simulink library "lib_fuel_converter"  (Simulink 4.00)
undefined symbols (not defined in the file): acc_mech_eff, acc_mech_pwr, acc_mech_trq, air_cp, amb_tmp, cyc_mph, ex_gas_cp, fc_acc_mass, fc_base_mass, fc_c2i_th_cond, fc_c_init_tmp, fc_cl2h_eff, fc_CO2_to_FUELgps, fc_cold, fc_cold_tmp, fc_cp, fc_ct_trq, fc_emisv, fc_ext_sarea, fc_fuel_den, fc_fuel_lhv, fc_h2x_th_cond, fc_h_air_flow, fc_h_cp, fc_h_init_tmp, fc_hood_emisv, fc_hood_sarea, fc_i2x_th_cond, fc_i_init_tmp, fc_inertia, fc_map_spd, fc_map_trq, fc_max_trq, fc_nn_model_name, fc_pwr_scale, fc_spd_scale, fc_trq_scale, fc_tstat, fc_x_init_tmp, fd_ratio, gb_num_init, gb_ratio, pow, vc_idle_spd, vc_key_on, veh_glider_mass, veh_mass, wh_radius
libraries: lib_fuel_converter x6, lib_etc x4
(part 3 of 4)

== system lib_fuel_converter/fuel converter  <fc> for series/spinning up or spinning down/effect of inertia (Nm) ==
  note: if initial speed is >0 and it is the
      | first time step ignore inertial loads
      | tm:2/6/01
  req'd spd (rad/s) : Inport  Port=1  LatchInput=off
  prev spd : Inport  Port=2  LatchInput=off
  Clock : Clock
      settings: DisplayTime=off  Decimation=10
  Constant : Constant  Value=fc_inertia
  Constant1 : Constant  Value=cyc_mph(1,2)
  Logical Operator : Logic  Operator=NAND  Inputs=2
  Logical Operator1 : Logic  Operator=NOT  Inputs=2
  Memory : Memory  X0=-0.1  InheritSampleTime=off
      settings: RTWStateStorageClass=Auto
  Memory1 : Memory  X0=0  InheritSampleTime=off
      settings: RTWStateStorageClass=Auto
  Product1 : Product  Inputs=**/*  Multiplication=Element-wise(.*)  SaturateOnIntegerOverflow=on
  Sum : Sum  Inputs=+-  SaturateOnIntegerOverflow=on
  Sum1 : Sum  Inputs=+-  SaturateOnIntegerOverflow=on
  (Nm) : Outport  Port=1  InitialOutput=0
  wires:
  Logical Operator1/1 -> Logical Operator/2
  Memory1/1 -> Logical Operator1/1
  Constant1/1 -> Logical Operator/1
  Logical Operator/1 -> Product1/4
  Sum/1 -> Product1/2
  Sum1/1 -> Product1/3
  req'd spd (rad/s)/1 -> Sum/1
  prev spd/1 -> Sum/2
  Product1/1 -> (Nm)/1
  Memory/1 -> Sum1/2
  Clock/1 -> Memory1/1, Memory/1, Sum1/1
  Constant/1 -> Product1/1

== system lib_fuel_converter/fuel converter  <fc> for series/spinning up or spinning down/just started spin-down/spin-up ==
  state : Inport  Port=1  LatchInput=off
  Logical Operator : Logic  Operator=AND  Inputs=2
  Logical Operator1 : Logic  Operator=NOT  Inputs=1
  Memory1 : Memory  X0=(cyc_mph(1,2)==0)  InheritSampleTime=off
      settings: RTWStateStorageClass=Auto
  trigger : Outport  Port=1  InitialOutput=0
  wires:
  Memory1/1 -> Logical Operator1/1
  Logical Operator1/1 -> Logical Operator/2
  Logical Operator/1 -> trigger/1
  state/1 -> Logical Operator/1, Memory1/1

== system lib_fuel_converter/fuel converter  <fc> for series/spinning up or spinning down/no-lag Reset Integrator ==
  in_1 : Inport  Port=1  LatchInput=off
  in_2 : Inport  Port=2  LatchInput=off
  in_3 : Inport  Port=3  LatchInput=off
  Constant : Constant  Value=0
  Memory : Memory  Orientation=left  X0=initval  InheritSampleTime=off
      settings: RTWStateStorageClass=Auto
  Product : Product  Inputs=2  Multiplication=Element-wise(.*)  SaturateOnIntegerOverflow=on
  Sum : Sum  Inputs=++  SaturateOnIntegerOverflow=on
  Switch : Switch  Threshold=eps
  dt : Subsystem  Orientation=down
      settings: RTWFcnNameOpts=Auto  RTWFileNameOpts=Auto
  in_2==0 : RelationalOperator  Operator===
  out_1 : Outport  Port=1  InitialOutput=0
  wires:
  in_3/1 -> Switch/3
  in_2/1 -> in_2==0/1
  in_1/1 -> Product/2
  dt/1(out_1) -> Product/1
  Product/1 -> Sum/2
  Memory/1 -> Sum/1
  Sum/1 -> Switch/1
  Switch/1 -> out_1/1, Memory/1
  in_2==0/1 -> Switch/2
  Constant/1 -> in_2==0/2

== system lib_fuel_converter/fuel converter  <fc> prius/providing trq (+ive or -ive)/accessories (Nm) ==
  w_APU : Inport  Port=1  LatchInput=off
  (Nm) : Product  Inputs=*/  Multiplication=Element-wise(.*)  SaturateOnIntegerOverflow=on
  (W) : Product  Inputs=*/  Multiplication=Element-wise(.*)  SaturateOnIntegerOverflow=on
  Constant : Constant  Value=acc_mech_pwr
  Constant1 : Constant  Value=acc_mech_eff
  Constant2 : Constant  Orientation=down  Value=acc_mech_trq
  Constant3 : Constant  Orientation=left  Value=0
  Saturation : Saturate  UpperLimit=inf  LowerLimit=vc_idle_spd+eps  LinearizeAsGain=on
  Sum : Sum  Inputs=++  SaturateOnIntegerOverflow=on
  Switch : Switch  Threshold=eps
  key_on : Subsystem  Orientation=left  mask(Repeating table){@1=vc_key_on(:,1), @2=vc_key_on(:,2)}
      mask prompts: @1 "Time values:"; @2 "Output values:"
      mask help:
      | Repeating table.
      | Enter values of time and output for first cycle.
      mask init:
      | period = max(@1); t = @1; y = @2;
      settings: RTWFcnNameOpts=Auto  RTWFileNameOpts=Auto
      mask Help: Repeats cycle given in table. Time values should be monotonically increasing.
  T_acc : Outport  Port=1  InitialOutput=0
  wires:
  Saturation/1 -> (Nm)/2
  Switch/1 -> T_acc/1
  Constant3/1 -> Switch/3
  key_on/1(out_1) -> Switch/2
  Sum/1 -> Switch/1
  Constant2/1 -> Sum/1
  (Nm)/1 -> Sum/2
  (W)/1 -> (Nm)/1
  w_APU/1 -> Saturation/1
  Constant1/1 -> (W)/2
  Constant/1 -> (W)/1

== system lib_fuel_converter/fuel converter  <fc> prius/providing trq (+ive or -ive)/effect of inertia (Nm) ==
  req'd spd (rad/s) : Inport  Port=1  LatchInput=off
  prev spd : Inport  Port=2  LatchInput=off
  Clock : Clock
      settings: DisplayTime=off  Decimation=10
  Constant : Constant  Value=fc_inertia
  Memory : Memory  X0=-0.1  InheritSampleTime=off
      settings: RTWStateStorageClass=Auto
  Product1 : Product  Inputs=**/  Multiplication=Element-wise(.*)  SaturateOnIntegerOverflow=on
  Sum : Sum  Inputs=+-  SaturateOnIntegerOverflow=on
  Sum1 : Sum  Inputs=+-  SaturateOnIntegerOverflow=on
  (Nm) : Outport  Port=1  InitialOutput=0
  wires:
  Sum/1 -> Product1/2
  Sum1/1 -> Product1/3
  req'd spd (rad/s)/1 -> Sum/1
  prev spd/1 -> Sum/2
  Product1/1 -> (Nm)/1
  Memory/1 -> Sum1/2
  Clock/1 -> Memory/1, Sum1/1
  Constant/1 -> Product1/1

== system lib_fuel_converter/fuel converter  <fc> prius/providing trq (+ive or -ive)/enforce engine limits ==
  req'd engine trq (Nm) : Inport  Port=1  LatchInput=off
  req'd engine spd (rad/s) : Inport  Port=2  LatchInput=off
  Block NOTES : Subsystem
      settings: RTWFcnNameOpts=Auto  RTWFileNameOpts=Auto
      mask Display: disp('Block\nNOTES')
  MinMax : MinMax  Function=min  Inputs=2
  MinMax1 : MinMax  Function=max  Inputs=2
  Relational Operator : RelationalOperator  Operator=~=
  Saturation : Saturate  UpperLimit=max(fc_map_spd)*fc_spd_scale  LowerLimit=0  LinearizeAsGain=on
  T_closed throttle : Subsystem
      settings: RTWFcnNameOpts=Auto  RTWFileNameOpts=Auto
  T_max : Subsystem
      settings: RTWFcnNameOpts=Auto  RTWFileNameOpts=Auto
  clutch disengaged1 : RelationalOperator  Operator=~=
  limited engine brake trq (Nm) : Outport  Port=1
  limited engine spd (rad/s) : Outport  Port=2
  tag scope: fc_spd_limited=global, fc_trq_limited=global
  wires:
  T_closed throttle/1(T_closed throttle) -> MinMax1/2
  Relational Operator/1 -> [fc_spd_limited]
  MinMax/1 -> MinMax1/1
  T_max/1(T_max) -> MinMax/2
  clutch disengaged1/1 -> [fc_trq_limited]
  MinMax1/1 -> limited engine brake trq (Nm)/1, clutch disengaged1/2
  req'd engine trq (Nm)/1 -> MinMax/1, clutch disengaged1/1
  Saturation/1 -> T_closed throttle/1(w_APU), T_max/1(w_APU), limited engine spd (rad/s)/1, Relational Operator/2
  req'd engine spd (rad/s)/1 -> Saturation/1, Relational Operator/1

== system lib_fuel_converter/configurable subsystems/fuel use and EO emis/HOT engine maps /Block NOTES ==
  note: This block determines the fully hot fuel use, engine-out emissions output rates, exhaust gas mass flow rate,
      | and engine-out exhaust gas temperature as a function of engine output torque and speed.
      | The engine maps (except for exhaust gas temperature) can be scaled using variables fc_spd_scale and
      |  fc_trq_scale; it is recommended that scaling values outside the range of 0.85 to 1.15 be used CAREFULLY.

== system lib_fuel_converter/configurable subsystems/fuel use and EO emis/HOT engine maps /CO (g/s) ==
  x0 : Inport  Port=1  LatchInput=off
  y0 : Inport  Port=2  LatchInput=off
  Mux : Mux  Inputs=2
      settings: DisplayOption=none
  S-function : S-Function  FunctionName=sftable2  Parameters=xindex, yindex, table  PortCounts=[]  SFunctionModules=''
  table out : Outport  Port=1  InitialOutput=0
  wires:
  y0/1 -> Mux/2
  S-function/1 -> table out/1
  x0/1 -> Mux/1
  Mux/1 -> S-function/1

== system lib_fuel_converter/configurable subsystems/fuel use and EO emis/HOT engine maps /HC (g/s) ==
  x0 : Inport  Port=1  LatchInput=off
  y0 : Inport  Port=2  LatchInput=off
  Mux : Mux  Inputs=2
      settings: DisplayOption=none
  S-function : S-Function  FunctionName=sftable2  Parameters=xindex, yindex, table  PortCounts=[]  SFunctionModules=''
  table out : Outport  Port=1  InitialOutput=0
  wires:
  y0/1 -> Mux/2
  S-function/1 -> table out/1
  x0/1 -> Mux/1
  Mux/1 -> S-function/1

== system lib_fuel_converter/configurable subsystems/fuel use and EO emis/HOT engine maps /MF,ex (g/s) ==
  x0 : Inport  Port=1  LatchInput=off
  y0 : Inport  Port=2  LatchInput=off
  Mux : Mux  Inputs=2
      settings: DisplayOption=none
  S-function : S-Function  FunctionName=sftable2  Parameters=xindex, yindex, table  PortCounts=[]  SFunctionModules=''
  table out : Outport  Port=1  InitialOutput=0
  wires:
  y0/1 -> Mux/2
  S-function/1 -> table out/1
  x0/1 -> Mux/1
  Mux/1 -> S-function/1

== system lib_fuel_converter/configurable subsystems/fuel use and EO emis/HOT engine maps /NOx (g/s) ==
  x0 : Inport  Port=1  LatchInput=off
  y0 : Inport  Port=2  LatchInput=off
  Mux : Mux  Inputs=2
      settings: DisplayOption=none
  S-function : S-Function  FunctionName=sftable2  Parameters=xindex, yindex, table  PortCounts=[]  SFunctionModules=''
  table out : Outport  Port=1  InitialOutput=0
  wires:
  y0/1 -> Mux/2
  S-function/1 -> table out/1
  x0/1 -> Mux/1
  Mux/1 -> S-function/1

== system lib_fuel_converter/configurable subsystems/fuel use and EO emis/HOT engine maps /O2 (g/s) ==
  x0 : Inport  Port=1  LatchInput=off
  y0 : Inport  Port=2  LatchInput=off
  Mux : Mux  Inputs=2
      settings: DisplayOption=none
  S-function : S-Function  FunctionName=sftable2  Parameters=xindex, yindex, table  PortCounts=[]  SFunctionModules=''
  table out : Outport  Port=1  InitialOutput=0
  wires:
  Mux/1 -> S-function/1
  x0/1 -> Mux/1
  S-function/1 -> table out/1
  y0/1 -> Mux/2

== system lib_fuel_converter/configurable subsystems/fuel use and EO emis/HOT engine maps /PM (g/s) ==
  x0 : Inport  Port=1  LatchInput=off
  y0 : Inport  Port=2  LatchInput=off
  Mux : Mux  Inputs=2
      settings: DisplayOption=none
  S-function : S-Function  FunctionName=sftable2  Parameters=xindex, yindex, table  PortCounts=[]  SFunctionModules=''
  table out : Outport  Port=1  InitialOutput=0
  wires:
  y0/1 -> Mux/2
  S-function/1 -> table out/1
  x0/1 -> Mux/1
  Mux/1 -> S-function/1

== system lib_fuel_converter/configurable subsystems/fuel use and EO emis/HOT engine maps /Tex,eo (C) ==
  x0 : Inport  Port=1  LatchInput=off
  y0 : Inport  Port=2  LatchInput=off
  Mux : Mux  Inputs=2
      settings: DisplayOption=none
  S-function : S-Function  FunctionName=sftable2  Parameters=xindex, yindex, table  PortCounts=[]  SFunctionModules=''
  table out : Outport  Port=1  InitialOutput=0
  wires:
  y0/1 -> Mux/2
  S-function/1 -> table out/1
  x0/1 -> Mux/1
  Mux/1 -> S-function/1

== system lib_fuel_converter/configurable subsystems/fuel use and EO emis/HOT engine maps /fuel (g/s) ==
  x0 : Inport  Port=1  LatchInput=off
  y0 : Inport  Port=2  LatchInput=off
  Mux : Mux  Inputs=2
      settings: DisplayOption=none
  S-function : S-Function  FunctionName=sftable2  Parameters=xindex, yindex, table  PortCounts=[]  SFunctionModules=''
  table out : Outport  Port=1  InitialOutput=0
  wires:
  y0/1 -> Mux/2
  S-function/1 -> table out/1
  x0/1 -> Mux/1
  Mux/1 -> S-function/1

== system lib_fuel_converter/configurable subsystems/fuel use and EO emis/fc temp/Block NOTES ==
  note: This block models the thermal behavior internal combustion engine (ICE).
      | Emphasis is on the coolant since this temperature is used to correct engine
      | fuel use.

== system lib_fuel_converter/configurable subsystems/fuel use and EO emis/fc temp/fc coolant ==
  Tcl : Inport  Port=1  LatchInput=off
  "Qfc_i " : Inport  Port=2  LatchInput=off
  Enable : EnablePort  StatesWhenEnabling=reset
  Constant : Constant  Value=fc_tstat
  Product1 : Product  Inputs=2  Multiplication=Element-wise(.*)  SaturateOnIntegerOverflow=on
  Qhtr : Fcn  Expr=fc_cl2h_eff*fc_h_air_flow*air_cp*(u - amb_tmp)
  Qi : Sum  Inputs=-+  SaturateOnIntegerOverflow=on
  Relational Operator : RelationalOperator  Operator=<=
  Qfc_rad : Outport  Port=1  OutputWhenDisabled=reset  InitialOutput=0
  Qfc_htr : Outport  Port=2  OutputWhenDisabled=reset  InitialOutput=0
  wires:
  Qi/1 -> Product1/2
  Qhtr/1 -> Qfc_htr/1, Qi/1
  "Qfc_i "/1 -> Qi/2
  Product1/1 -> Qfc_rad/1
  Constant/1 -> Relational Operator/1
  Relational Operator/1 -> Product1/1
  Tcl/1 -> Relational Operator/2, Qhtr/1

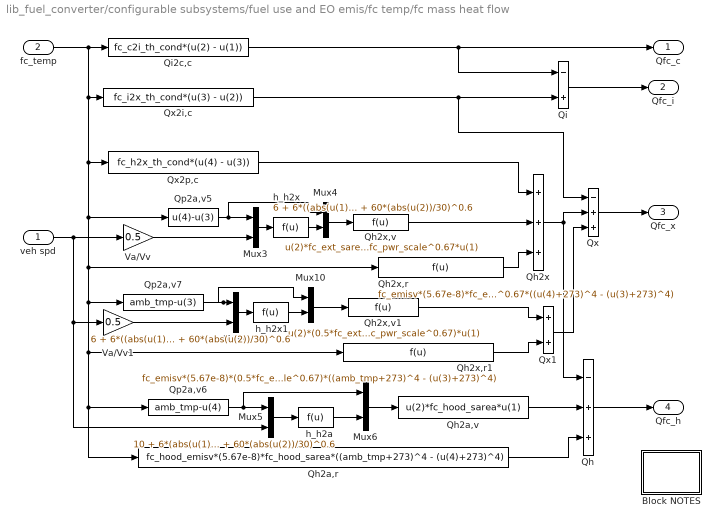
== system lib_fuel_converter/configurable subsystems/fuel use and EO emis/fc temp/fc mass heat flow ==
  veh spd : Inport  Port=1  LatchInput=off
  fc_temp : Inport  Port=2  LatchInput=off
  Block NOTES : Subsystem
      settings: RTWFcnNameOpts=Auto  RTWFileNameOpts=Auto
      mask Display: disp('Block\nNOTES')
  Mux{3..6,9..10} (6 alike) : Mux  Inputs=2
      settings: DisplayOption=none
  Qh : Sum  Inputs=-++  SaturateOnIntegerOverflow=on
  Qh2a,r : Fcn  Expr=fc_hood_emisv*(5.67e-8)*fc_hood_sarea*((amb_tmp+273)^4 - (u(4)+273)^4)
  Qh2a,v : Fcn  Expr=u(2)*fc_hood_sarea*u(1)
  Qh2x : Sum  Inputs=+++  SaturateOnIntegerOverflow=on
  Qh2x,r : Fcn  Expr=fc_emisv*(5.67e-8)*fc_ext_sarea*fc_pwr_scale^0.67*((u(4)+273)^4 - (u(3)+273)^4)
  Qh2x,r1 : Fcn  Expr=fc_emisv*(5.67e-8)*(0.5*fc_ext_sarea*fc_pwr_scale^0.67)*((amb_tmp+273)^4 - (u(3)+273)^4)
  Qh2x,v : Fcn  Expr=u(2)*fc_ext_sarea*fc_pwr_scale^0.67*u(1)
  Qh2x,v1 : Fcn  Expr=u(2)*(0.5*fc_ext_sarea*fc_pwr_scale^0.67)*u(1)
  Qi : Sum  Inputs=-+  SaturateOnIntegerOverflow=on
  Qi2c,c : Fcn  Expr=fc_c2i_th_cond*(u(2) - u(1))
  Qp2a,v5 : Fcn  Expr=u(4)-u(3)
  Qp2a,v6 : Fcn  Expr=amb_tmp-u(4)
  Qp2a,v7 : Fcn  Expr=amb_tmp-u(3)
  Qx : Sum  Inputs=-++  SaturateOnIntegerOverflow=on
  Qx1 : Sum  Inputs=++  SaturateOnIntegerOverflow=on
  Qx2i,c : Fcn  Expr=fc_i2x_th_cond*(u(3) - u(2))
  Qx2p,c : Fcn  Expr=fc_h2x_th_cond*(u(4) - u(3))
  Va/Vv : Gain  Gain=0.5  Multiplication=Element-wise(K.*u)  SaturateOnIntegerOverflow=on
  Va/Vv1 : Gain  Gain=0.5  Multiplication=Element-wise(K.*u)  SaturateOnIntegerOverflow=on
  h_h2a : Fcn  Expr=10 + 6*(abs(u(1))/1000)^0.3 + 60*(abs(u(2))/30)^0.6
  h_h2x : Fcn  Expr=6 + 6*((abs(u(1))/1000))^0.3 + 60*(abs(u(2))/30)^0.6
  h_h2x1 : Fcn  Expr=6 + 6*((abs(u(1))/1000))^0.3 + 60*(abs(u(2))/30)^0.6
  Qfc_c : Outport  Port=1
  Qfc_i : Outport  Port=2
  Qfc_x : Outport  Port=3
  Qfc_h : Outport  Port=4
  wires:
  Qh2x,r/1 -> Qh2x/3
  Qh2a,v/1 -> Qh/2
  Qh2a,r/1 -> Qh/3
  Qh2x,v1/1 -> Qx1/1
  Qh2x,r1/1 -> Qx1/2
  Qx2p,c/1 -> Qh2x/1
  Qh2x,v/1 -> Qh2x/2
  Qx1/1 -> Qx/3
  h_h2a/1 -> Mux6/2
  Qp2a,v6/1 -> Mux6/1, Mux5/1
  Mux5/1 -> h_h2a/1
  Mux6/1 -> Qh2a,v/1
  Qh/1 -> Qfc_h/1
  Qh2x/1 -> Qh/1, Qx/2
  Qx/1 -> Qfc_x/1
  Qi/1 -> Qfc_i/1
  Qx2i,c/1 -> Qx/1, Qi/2
  fc_temp/1 -> Qi2c,c/1, Qx2i,c/1, Qp2a,v5/1, Qh2x,r1/1, Qh2a,r/1, Qp2a,v6/1, Qp2a,v7/1, Qh2x,r/1, Qx2p,c/1
  Qi2c,c/1 -> Qi/1, Qfc_c/1
  Va/Vv/1 -> Mux3/2
  veh spd/1 -> Va/Vv1/1, Mux5/2, Va/Vv/1
  h_h2x/1 -> Mux4/2
  Qp2a,v5/1 -> Mux4/1, Mux3/1
  Mux3/1 -> h_h2x/1
  Mux4/1 -> Qh2x,v/1
  Va/Vv1/1 -> Mux9/2
  h_h2x1/1 -> Mux10/2
  Qp2a,v7/1 -> Mux10/1, Mux9/1
  Mux9/1 -> h_h2x1/1
  Mux10/1 -> Qh2x,v1/1

== system lib_fuel_converter/configurable subsystems/fuel use and EO emis/fc temp/old fc coolant  temp. (C) ==
  fc on? : Inport  Port=1  LatchInput=off
  veh spd : Inport  Port=2  LatchInput=off
  Block NOTES : Subsystem
      settings: RTWFcnNameOpts=Auto  RTWFileNameOpts=Auto
      mask Display: disp('Block\nNOTES')
  Mux : Mux  Inputs=4
      settings: DisplayOption=none
  TEC : Integrator  ExternalReset=none  InitialConditionSource=internal  InitialCondition=fc_i_init_tmp  LimitOutput=off  UpperSaturationLimit=inf  LowerSaturationLimit=-inf  ShowSaturationPort=off  ShowStatePort=off  AbsoluteTolerance=auto
  compute engine dT/dt : Fcn  Expr=1.1*u[1]*(-u[2]/218)*(95-u[4])+(1-u[1])*u[3]*(u[4]-amb_tmp)
  gamma (takes v as input) : Fcn  Expr=(-8.22e-5*u+8.09e-6*4-1.45e-4)*.45
  log(1-40/75) : Constant  Value=-0.7621
  fc coolant  temp (C) : Outport  Port=1  InitialOutput=0
  wires:
  TEC/1 -> Mux/4, fc coolant  temp (C)/1
  veh spd/1 -> gamma (takes v as input)/1
  fc on?/1 -> Mux/1
  Mux/1 -> compute engine dT/dt/1
  log(1-40/75)/1 -> Mux/2
  gamma (takes v as input)/1 -> Mux/3
  compute engine dT/dt/1 -> TEC/1

== system lib_fuel_converter/configurable subsystems/fuel use and EO emis/fc temp correct/fc temp correct Constant Correction Factors (Equation Based) ==
  Coolant T (C) : Inport  Port=1  LatchInput=off
  HOT fuel use (g/s) : Inport  Port=2  LatchInput=off
  HOT emis (g/s) : Inport  Port=3  LatchInput=off
  Enable : EnablePort  StatesWhenEnabling=reset
  Block NOTES : Subsystem
      settings: RTWFcnNameOpts=Auto  RTWFileNameOpts=Auto
      mask Display: disp('Block\nNOTES')
  CO cold/hot : Fcn  Expr=2.13*pow(u,4.26)+1
  HC cold/hot : Fcn  Expr=8.05*pow(u,9.46)+1
  Mux : Mux  Inputs=4
      settings: DisplayOption=none
  NOx cold/hot : Fcn  Expr=0.51*pow(u,1.37)+1
  PM cold/hot : Fcn  Expr=5.14*pow(u,17.04)+1
  Product : Product  Inputs=2  Multiplication=Element-wise(.*)  SaturateOnIntegerOverflow=on
  Product1 : Product  Inputs=2  Multiplication=Element-wise(.*)  SaturateOnIntegerOverflow=on
  Saturation : Saturate  UpperLimit=1  LowerLimit=0  LinearizeAsGain=on
  fuel cold/hot : Fcn  Expr=0.1*pow(u,0.65)+1
  lambda : Fcn  Expr=(fc_tstat-u)/(fc_tstat-20)
  fuel use (g/s) : Outport  Port=1  OutputWhenDisabled=reset  InitialOutput=0
  EO emis (g/s) : Outport  Port=2  OutputWhenDisabled=reset  InitialOutput=0
  wires:
  HOT emis (g/s)/1 -> Product/2
  Coolant T (C)/1 -> lambda/1
  HOT fuel use (g/s)/1 -> Product1/1
  Product1/1 -> fuel use (g/s)/1
  CO cold/hot/1 -> Mux/2
  Product/1 -> EO emis (g/s)/1
  fuel cold/hot/1 -> Product1/2
  Mux/1 -> Product/1
  lambda/1 -> Saturation/1
  Saturation/1 -> PM cold/hot/1, NOx cold/hot/1, fuel cold/hot/1, HC cold/hot/1, CO cold/hot/1
  HC cold/hot/1 -> Mux/1
  NOx cold/hot/1 -> Mux/3
  PM cold/hot/1 -> Mux/4

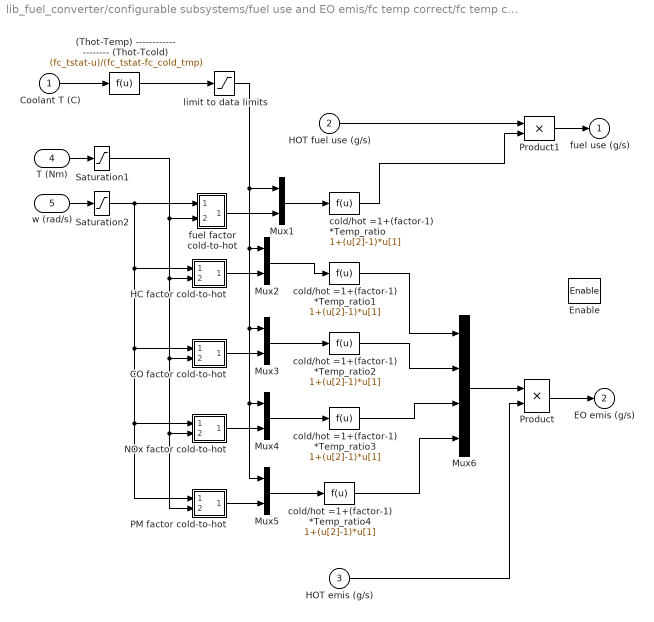
== system lib_fuel_converter/configurable subsystems/fuel use and EO emis/fc temp correct/fc temp correct Variable Correction Factors (Map Based) ==
  Coolant T (C) : Inport  Port=1  LatchInput=off
  HOT fuel use (g/s) : Inport  Port=2  LatchInput=off
  HOT emis (g/s) : Inport  Port=3  LatchInput=off
  T (Nm) : Inport  Port=4  LatchInput=off
  w (rad/s) : Inport  Port=5  LatchInput=off
  Enable : EnablePort  StatesWhenEnabling=reset
  (Thot-Temp) -------------------- (Thot-Tcold) : Fcn  Expr=(fc_tstat-u)/(fc_tstat-fc_cold_tmp)
  CO factor cold-to-hot : Subsystem  mask(2-D Table Lookup){@1=fc_map_spd*fc_spd_scale, @2=fc_map_trq*fc_trq_scale, @3=fc_co_map_c2h}
      mask prompts: @1 "X Index"; @2 "Y Index"; @3 "Table"
      mask help:
      | Two Dimensional Table Lookup
      | The first input corresponds to X Index and the second input corresponds to the Y Index
      mask init:
      | xindex=@1; yindex=@2; table=@3; sftab2chk(xindex,yindex,table);
      settings: RTWFcnNameOpts=Auto  RTWFileNameOpts=Auto
      mask Help: This block returns a linearly interpolated intersection from the table using the X index (which corresponds to the rows of the table) and the Y index (which corresponds to the columns of the table).  Extrapolation is used.
      mask Display: plot(-10,-10,110,110,[90,50,10],[90,40,30],[90,50,10],[50,26,20],[90,50,10],[22,13,10])
  HC factor cold-to-hot : Subsystem  mask(2-D Table Lookup){@1=fc_map_spd*fc_spd_scale, @2=fc_map_trq*fc_trq_scale, @3=fc_hc_map_c2h}
      mask prompts: @1 "X Index"; @2 "Y Index"; @3 "Table"
      mask help:
      | Two Dimensional Table Lookup
      | The first input corresponds to X Index and the second input corresponds to the Y Index
      mask init:
      | xindex=@1; yindex=@2; table=@3; sftab2chk(xindex,yindex,table);
      settings: RTWFcnNameOpts=Auto  RTWFileNameOpts=Auto
      mask Help: This block returns a linearly interpolated intersection from the table using the X index (which corresponds to the rows of the table) and the Y index (which corresponds to the columns of the table).  Extrapolation is used.
      mask Display: plot(-10,-10,110,110,[90,50,10],[90,40,30],[90,50,10],[50,26,20],[90,50,10],[22,13,10])
  Mux{1..5} (5 alike) : Mux  Inputs=2
      settings: DisplayOption=none
  Mux6 : Mux  Inputs=4
      settings: DisplayOption=none
  NOx factor cold-to-hot : Subsystem  mask(2-D Table Lookup){@1=fc_map_spd*fc_spd_scale, @2=fc_map_trq*fc_trq_scale, @3=fc_nox_map_c2h}
      mask prompts: @1 "X Index"; @2 "Y Index"; @3 "Table"
      mask help:
      | Two Dimensional Table Lookup
      | The first input corresponds to X Index and the second input corresponds to the Y Index
      mask init:
      | xindex=@1; yindex=@2; table=@3; sftab2chk(xindex,yindex,table);
      settings: RTWFcnNameOpts=Auto  RTWFileNameOpts=Auto
      mask Help: This block returns a linearly interpolated intersection from the table using the X index (which corresponds to the rows of the table) and the Y index (which corresponds to the columns of the table).  Extrapolation is used.
      mask Display: plot(-10,-10,110,110,[90,50,10],[90,40,30],[90,50,10],[50,26,20],[90,50,10],[22,13,10])
  PM factor cold-to-hot : Subsystem  mask(2-D Table Lookup){@1=fc_map_spd*fc_spd_scale, @2=fc_map_trq*fc_trq_scale, @3=fc_pm_map_c2h}
      mask prompts: @1 "X Index"; @2 "Y Index"; @3 "Table"
      mask help:
      | Two Dimensional Table Lookup
      | The first input corresponds to X Index and the second input corresponds to the Y Index
      mask init:
      | xindex=@1; yindex=@2; table=@3; sftab2chk(xindex,yindex,table);
      settings: RTWFcnNameOpts=Auto  RTWFileNameOpts=Auto
      mask Help: This block returns a linearly interpolated intersection from the table using the X index (which corresponds to the rows of the table) and the Y index (which corresponds to the columns of the table).  Extrapolation is used.
      mask Display: plot(-10,-10,110,110,[90,50,10],[90,40,30],[90,50,10],[50,26,20],[90,50,10],[22,13,10])
  Product : Product  Inputs=2  Multiplication=Element-wise(.*)  SaturateOnIntegerOverflow=on
  Product1 : Product  Inputs=2  Multiplication=Element-wise(.*)  SaturateOnIntegerOverflow=on
  Saturation1 : Saturate  UpperLimit=max(fc_map_trq*fc_trq_scale)  LowerLimit=min(fc_map_trq*fc_trq_scale)  LinearizeAsGain=on
  Saturation2 : Saturate  UpperLimit=max(fc_map_spd*fc_spd_scale)  LowerLimit=min(fc_map_spd*fc_spd_scale)  LinearizeAsGain=on
  cold/hot =1+(factor-1) *Temp_ratio{,1..4} (5 alike) : Fcn  Expr=1+(u[2]-1)*u[1]
  fuel factor cold-to-hot : Subsystem  mask(2-D Table Lookup){@1=fc_map_spd*fc_spd_scale, @2=fc_map_trq*fc_trq_scale, @3=fc_fuel_map_c2h}
      mask prompts: @1 "X Index"; @2 "Y Index"; @3 "Table"
      mask help:
      | Two Dimensional Table Lookup
      | The first input corresponds to X Index and the second input corresponds to the Y Index
      mask init:
      | xindex=@1; yindex=@2; table=@3; sftab2chk(xindex,yindex,table);
      settings: RTWFcnNameOpts=Auto  RTWFileNameOpts=Auto
      mask Help: This block returns a linearly interpolated intersection from the table using the X index (which corresponds to the rows of the table) and the Y index (which corresponds to the columns of the table).  Extrapolation is used.
      mask Display: plot(-10,-10,110,110,[90,50,10],[90,40,30],[90,50,10],[50,26,20],[90,50,10],[22,13,10])
  limit to data limits : Saturate  UpperLimit=1  LowerLimit=0  LinearizeAsGain=on
  fuel use (g/s) : Outport  Port=1  OutputWhenDisabled=reset  InitialOutput=0
  EO emis (g/s) : Outport  Port=2  OutputWhenDisabled=reset  InitialOutput=0
  wires:
  HOT fuel use (g/s)/1 -> Product1/1
  Saturation2/1 -> fuel factor cold-to-hot/1(x0), HC factor cold-to-hot/1(x0), CO factor cold-to-hot/1(x0), NOx factor cold-to-hot/1(x0), PM factor cold-to-hot/1(x0)
  Saturation1/1 -> fuel factor cold-to-hot/2(y0), HC factor cold-to-hot/2(y0), CO factor cold-to-hot/2(y0), NOx factor cold-to-hot/2(y0), PM factor cold-to-hot/2(y0)
  Coolant T (C)/1 -> (Thot-Temp) -------------------- (Thot-Tcold)/1
  fuel factor cold-to-hot/1(table out) -> Mux1/2
  Mux1/1 -> cold/hot =1+(factor-1) *Temp_ratio/1
  HC factor cold-to-hot/1(table out) -> Mux2/2
  CO factor cold-to-hot/1(table out) -> Mux3/2
  NOx factor cold-to-hot/1(table out) -> Mux4/2
  PM factor cold-to-hot/1(table out) -> Mux5/2
  Mux2/1 -> cold/hot =1+(factor-1) *Temp_ratio1/1
  Mux3/1 -> cold/hot =1+(factor-1) *Temp_ratio2/1
  Mux4/1 -> cold/hot =1+(factor-1) *Temp_ratio3/1
  Mux5/1 -> cold/hot =1+(factor-1) *Temp_ratio4/1
  Product1/1 -> fuel use (g/s)/1
  Product/1 -> EO emis (g/s)/1
  HOT emis (g/s)/1 -> Product/2
  T (Nm)/1 -> Saturation1/1
  w (rad/s)/1 -> Saturation2/1
  Mux6/1 -> Product/1
  (Thot-Temp) -------------------- (Thot-Tcold)/1 -> limit to data limits/1
  limit to data limits/1 -> Mux1/1, Mux2/1, Mux3/1, Mux4/1, Mux5/1
  cold/hot =1+(factor-1) *Temp_ratio/1 -> Product1/2
  cold/hot =1+(factor-1) *Temp_ratio1/1 -> Mux6/1
  cold/hot =1+(factor-1) *Temp_ratio2/1 -> Mux6/2
  cold/hot =1+(factor-1) *Temp_ratio3/1 -> Mux6/3
  cold/hot =1+(factor-1) *Temp_ratio4/1 -> Mux6/4

== system lib_fuel_converter/configurable subsystems/fuel use and EO emis Neural Network Model/HOT engine maps /Block NOTES ==
  note: This block determines the fully hot fuel use, engine-out emissions output rates, exhaust gas mass flow rate,
      | and engine-out exhaust gas temperature as a function of engine output torque and speed.
      | The engine maps (except for exhaust gas temperature) can be scaled using variables fc_spd_scale and
      |  fc_trq_scale; it is recommended that scaling values outside the range of 0.85 to 1.15 be used CAREFULLY.

== system lib_fuel_converter/configurable subsystems/fuel use and EO emis Neural Network Model/HOT engine maps /CO (g/s) ==
  x0 : Inport  Port=1  LatchInput=off
  y0 : Inport  Port=2  LatchInput=off
  Mux : Mux  Inputs=2
      settings: DisplayOption=none
  S-function : S-Function  FunctionName=sftable2  Parameters=xindex, yindex, table  PortCounts=[]  SFunctionModules=''
  table out : Outport  Port=1  InitialOutput=0
  wires:
  y0/1 -> Mux/2
  S-function/1 -> table out/1
  x0/1 -> Mux/1
  Mux/1 -> S-function/1

== system lib_fuel_converter/configurable subsystems/fuel use and EO emis Neural Network Model/HOT engine maps /HC (g/s) ==
  x0 : Inport  Port=1  LatchInput=off
  y0 : Inport  Port=2  LatchInput=off
  Mux : Mux  Inputs=2
      settings: DisplayOption=none
  S-function : S-Function  FunctionName=sftable2  Parameters=xindex, yindex, table  PortCounts=[]  SFunctionModules=''
  table out : Outport  Port=1  InitialOutput=0
  wires:
  y0/1 -> Mux/2
  S-function/1 -> table out/1
  x0/1 -> Mux/1
  Mux/1 -> S-function/1

== system lib_fuel_converter/configurable subsystems/fuel use and EO emis Neural Network Model/HOT engine maps /MF,ex (g/s) ==
  x0 : Inport  Port=1  LatchInput=off
  y0 : Inport  Port=2  LatchInput=off
  Mux : Mux  Inputs=2
      settings: DisplayOption=none
  S-function : S-Function  FunctionName=sftable2  Parameters=xindex, yindex, table  PortCounts=[]  SFunctionModules=''
  table out : Outport  Port=1  InitialOutput=0
  wires:
  y0/1 -> Mux/2
  S-function/1 -> table out/1
  x0/1 -> Mux/1
  Mux/1 -> S-function/1

== system lib_fuel_converter/configurable subsystems/fuel use and EO emis Neural Network Model/HOT engine maps /NOx (g/s) ==
  x0 : Inport  Port=1  LatchInput=off
  y0 : Inport  Port=2  LatchInput=off
  Mux : Mux  Inputs=2
      settings: DisplayOption=none
  S-function : S-Function  FunctionName=sftable2  Parameters=xindex, yindex, table  PortCounts=[]  SFunctionModules=''
  table out : Outport  Port=1  InitialOutput=0
  wires:
  y0/1 -> Mux/2
  S-function/1 -> table out/1
  x0/1 -> Mux/1
  Mux/1 -> S-function/1

== system lib_fuel_converter/configurable subsystems/fuel use and EO emis Neural Network Model/HOT engine maps /O2 (g/s) ==
  x0 : Inport  Port=1  LatchInput=off
  y0 : Inport  Port=2  LatchInput=off
  Mux : Mux  Inputs=2
      settings: DisplayOption=none
  S-function : S-Function  FunctionName=sftable2  Parameters=xindex, yindex, table  PortCounts=[]  SFunctionModules=''
  table out : Outport  Port=1  InitialOutput=0
  wires:
  Mux/1 -> S-function/1
  x0/1 -> Mux/1
  S-function/1 -> table out/1
  y0/1 -> Mux/2

== system lib_fuel_converter/configurable subsystems/fuel use and EO emis Neural Network Model/HOT engine maps /PM (g/s) ==
  x0 : Inport  Port=1  LatchInput=off
  y0 : Inport  Port=2  LatchInput=off
  Mux : Mux  Inputs=2
      settings: DisplayOption=none
  S-function : S-Function  FunctionName=sftable2  Parameters=xindex, yindex, table  PortCounts=[]  SFunctionModules=''
  table out : Outport  Port=1  InitialOutput=0
  wires:
  y0/1 -> Mux/2
  S-function/1 -> table out/1
  x0/1 -> Mux/1
  Mux/1 -> S-function/1

== system lib_fuel_converter/configurable subsystems/fuel use and EO emis Neural Network Model/HOT engine maps /Tex,eo (C) ==
  x0 : Inport  Port=1  LatchInput=off
  y0 : Inport  Port=2  LatchInput=off
  Mux : Mux  Inputs=2
      settings: DisplayOption=none
  S-function : S-Function  FunctionName=sftable2  Parameters=xindex, yindex, table  PortCounts=[]  SFunctionModules=''
  table out : Outport  Port=1  InitialOutput=0
  wires:
  y0/1 -> Mux/2
  S-function/1 -> table out/1
  x0/1 -> Mux/1
  Mux/1 -> S-function/1

== system lib_fuel_converter/configurable subsystems/fuel use and EO emis Neural Network Model/HOT engine maps /fuel (g/s) ==
  x0 : Inport  Port=1  LatchInput=off
  y0 : Inport  Port=2  LatchInput=off
  Mux : Mux  Inputs=2
      settings: DisplayOption=none
  S-function : S-Function  FunctionName=sftable2  Parameters=xindex, yindex, table  PortCounts=[]  SFunctionModules=''
  table out : Outport  Port=1  InitialOutput=0
  wires:
  y0/1 -> Mux/2
  S-function/1 -> table out/1
  x0/1 -> Mux/1
  Mux/1 -> S-function/1

== system lib_fuel_converter/configurable subsystems/fuel use and EO emis Neural Network Model/fc temp/Block NOTES ==
  note: This block models the thermal behavior internal combustion engine (ICE).
      | Emphasis is on the coolant since this temperature is used to correct engine
      | fuel use.

== system lib_fuel_converter/configurable subsystems/fuel use and EO emis Neural Network Model/fc temp/fc coolant ==
  Tcl : Inport  Port=1  LatchInput=off
  "Qfc_i " : Inport  Port=2  LatchInput=off
  Enable : EnablePort  StatesWhenEnabling=reset
  Constant : Constant  Value=fc_tstat
  Product1 : Product  Inputs=2  Multiplication=Element-wise(.*)  SaturateOnIntegerOverflow=on
  Qhtr : Fcn  Expr=fc_cl2h_eff*fc_h_air_flow*air_cp*(u - amb_tmp)
  Qi : Sum  Inputs=-+  SaturateOnIntegerOverflow=on
  Relational Operator : RelationalOperator  Operator=<=
  Qfc_rad : Outport  Port=1  OutputWhenDisabled=reset  InitialOutput=0
  Qfc_htr : Outport  Port=2  OutputWhenDisabled=reset  InitialOutput=0
  wires:
  Qi/1 -> Product1/2
  Qhtr/1 -> Qfc_htr/1, Qi/1
  "Qfc_i "/1 -> Qi/2
  Product1/1 -> Qfc_rad/1
  Constant/1 -> Relational Operator/1
  Relational Operator/1 -> Product1/1
  Tcl/1 -> Relational Operator/2, Qhtr/1

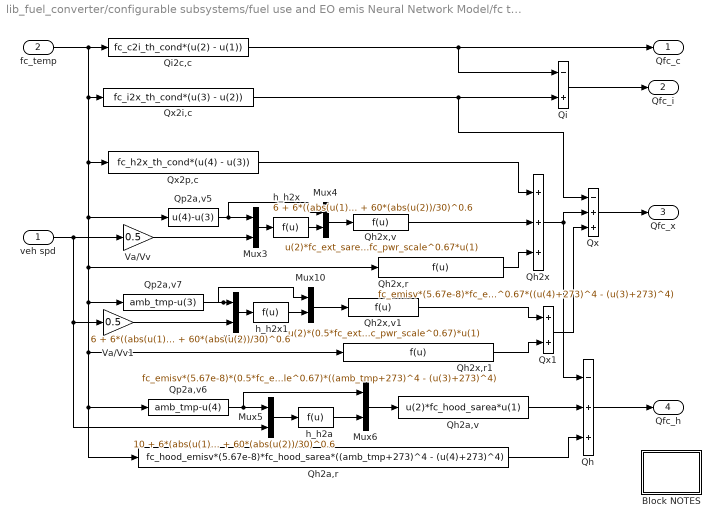
== system lib_fuel_converter/configurable subsystems/fuel use and EO emis Neural Network Model/fc temp/fc mass heat flow ==
  veh spd : Inport  Port=1  LatchInput=off
  fc_temp : Inport  Port=2  LatchInput=off
  Block NOTES : Subsystem
      settings: RTWFcnNameOpts=Auto  RTWFileNameOpts=Auto
      mask Display: disp('Block\nNOTES')
  Mux{3..6,9..10} (6 alike) : Mux  Inputs=2
      settings: DisplayOption=none
  Qh : Sum  Inputs=-++  SaturateOnIntegerOverflow=on
  Qh2a,r : Fcn  Expr=fc_hood_emisv*(5.67e-8)*fc_hood_sarea*((amb_tmp+273)^4 - (u(4)+273)^4)
  Qh2a,v : Fcn  Expr=u(2)*fc_hood_sarea*u(1)
  Qh2x : Sum  Inputs=+++  SaturateOnIntegerOverflow=on
  Qh2x,r : Fcn  Expr=fc_emisv*(5.67e-8)*fc_ext_sarea*fc_pwr_scale^0.67*((u(4)+273)^4 - (u(3)+273)^4)
  Qh2x,r1 : Fcn  Expr=fc_emisv*(5.67e-8)*(0.5*fc_ext_sarea*fc_pwr_scale^0.67)*((amb_tmp+273)^4 - (u(3)+273)^4)
  Qh2x,v : Fcn  Expr=u(2)*fc_ext_sarea*fc_pwr_scale^0.67*u(1)
  Qh2x,v1 : Fcn  Expr=u(2)*(0.5*fc_ext_sarea*fc_pwr_scale^0.67)*u(1)
  Qi : Sum  Inputs=-+  SaturateOnIntegerOverflow=on
  Qi2c,c : Fcn  Expr=fc_c2i_th_cond*(u(2) - u(1))
  Qp2a,v5 : Fcn  Expr=u(4)-u(3)
  Qp2a,v6 : Fcn  Expr=amb_tmp-u(4)
  Qp2a,v7 : Fcn  Expr=amb_tmp-u(3)
  Qx : Sum  Inputs=-++  SaturateOnIntegerOverflow=on
  Qx1 : Sum  Inputs=++  SaturateOnIntegerOverflow=on
  Qx2i,c : Fcn  Expr=fc_i2x_th_cond*(u(3) - u(2))
  Qx2p,c : Fcn  Expr=fc_h2x_th_cond*(u(4) - u(3))
  Va/Vv : Gain  Gain=0.5  Multiplication=Element-wise(K.*u)  SaturateOnIntegerOverflow=on
  Va/Vv1 : Gain  Gain=0.5  Multiplication=Element-wise(K.*u)  SaturateOnIntegerOverflow=on
  h_h2a : Fcn  Expr=10 + 6*(abs(u(1))/1000)^0.3 + 60*(abs(u(2))/30)^0.6
  h_h2x : Fcn  Expr=6 + 6*((abs(u(1))/1000))^0.3 + 60*(abs(u(2))/30)^0.6
  h_h2x1 : Fcn  Expr=6 + 6*((abs(u(1))/1000))^0.3 + 60*(abs(u(2))/30)^0.6
  Qfc_c : Outport  Port=1
  Qfc_i : Outport  Port=2
  Qfc_x : Outport  Port=3
  Qfc_h : Outport  Port=4
  wires:
  Qh2x,r/1 -> Qh2x/3
  Qh2a,v/1 -> Qh/2
  Qh2a,r/1 -> Qh/3
  Qh2x,v1/1 -> Qx1/1
  Qh2x,r1/1 -> Qx1/2
  Qx2p,c/1 -> Qh2x/1
  Qh2x,v/1 -> Qh2x/2
  Qx1/1 -> Qx/3
  h_h2a/1 -> Mux6/2
  Qp2a,v6/1 -> Mux6/1, Mux5/1
  Mux5/1 -> h_h2a/1
  Mux6/1 -> Qh2a,v/1
  Qh/1 -> Qfc_h/1
  Qh2x/1 -> Qh/1, Qx/2
  Qx/1 -> Qfc_x/1
  Qi/1 -> Qfc_i/1
  Qx2i,c/1 -> Qx/1, Qi/2
  fc_temp/1 -> Qi2c,c/1, Qx2i,c/1, Qp2a,v5/1, Qh2x,r1/1, Qh2a,r/1, Qp2a,v6/1, Qp2a,v7/1, Qh2x,r/1, Qx2p,c/1
  Qi2c,c/1 -> Qi/1, Qfc_c/1
  Va/Vv/1 -> Mux3/2
  veh spd/1 -> Va/Vv1/1, Mux5/2, Va/Vv/1
  h_h2x/1 -> Mux4/2
  Qp2a,v5/1 -> Mux4/1, Mux3/1
  Mux3/1 -> h_h2x/1
  Mux4/1 -> Qh2x,v/1
  Va/Vv1/1 -> Mux9/2
  h_h2x1/1 -> Mux10/2
  Qp2a,v7/1 -> Mux10/1, Mux9/1
  Mux9/1 -> h_h2x1/1
  Mux10/1 -> Qh2x,v1/1

== system lib_fuel_converter/configurable subsystems/fuel use and EO emis Neural Network Model/fc temp/old fc coolant  temp. (C) ==
  fc on? : Inport  Port=1  LatchInput=off
  veh spd : Inport  Port=2  LatchInput=off
  Block NOTES : Subsystem
      settings: RTWFcnNameOpts=Auto  RTWFileNameOpts=Auto
      mask Display: disp('Block\nNOTES')
  Mux : Mux  Inputs=4
      settings: DisplayOption=none
  TEC : Integrator  ExternalReset=none  InitialConditionSource=internal  InitialCondition=fc_i_init_tmp  LimitOutput=off  UpperSaturationLimit=inf  LowerSaturationLimit=-inf  ShowSaturationPort=off  ShowStatePort=off  AbsoluteTolerance=auto
  compute engine dT/dt : Fcn  Expr=1.1*u[1]*(-u[2]/218)*(95-u[4])+(1-u[1])*u[3]*(u[4]-amb_tmp)
  gamma (takes v as input) : Fcn  Expr=(-8.22e-5*u+8.09e-6*4-1.45e-4)*.45
  log(1-40/75) : Constant  Value=-0.7621
  fc coolant  temp (C) : Outport  Port=1  InitialOutput=0
  wires:
  TEC/1 -> Mux/4, fc coolant  temp (C)/1
  veh spd/1 -> gamma (takes v as input)/1
  fc on?/1 -> Mux/1
  Mux/1 -> compute engine dT/dt/1
  log(1-40/75)/1 -> Mux/2
  gamma (takes v as input)/1 -> Mux/3
  compute engine dT/dt/1 -> TEC/1

== system lib_fuel_converter/configurable subsystems/fuel use and EO emis Neural Network Model/fc temp correct/fc temp correct Constant Correction Factors (Equation Based) ==
  Coolant T (C) : Inport  Port=1  LatchInput=off
  HOT fuel use (g/s) : Inport  Port=2  LatchInput=off
  HOT emis (g/s) : Inport  Port=3  LatchInput=off
  Enable : EnablePort  StatesWhenEnabling=reset
  Block NOTES : Subsystem
      settings: RTWFcnNameOpts=Auto  RTWFileNameOpts=Auto
      mask Display: disp('Block\nNOTES')
  CO cold/hot : Fcn  Expr=2.13*pow(u,4.26)+1
  HC cold/hot : Fcn  Expr=8.05*pow(u,9.46)+1
  Mux : Mux  Inputs=4
      settings: DisplayOption=none
  NOx cold/hot : Fcn  Expr=0.51*pow(u,1.37)+1
  PM cold/hot : Fcn  Expr=5.14*pow(u,17.04)+1
  Product : Product  Inputs=2  Multiplication=Element-wise(.*)  SaturateOnIntegerOverflow=on
  Product1 : Product  Inputs=2  Multiplication=Element-wise(.*)  SaturateOnIntegerOverflow=on
  Saturation : Saturate  UpperLimit=1  LowerLimit=0  LinearizeAsGain=on
  fuel cold/hot : Fcn  Expr=0.1*pow(u,0.65)+1
  lambda : Fcn  Expr=(fc_tstat-u)/(fc_tstat-20)
  fuel use (g/s) : Outport  Port=1  OutputWhenDisabled=reset  InitialOutput=0
  EO emis (g/s) : Outport  Port=2  OutputWhenDisabled=reset  InitialOutput=0
  wires:
  HOT emis (g/s)/1 -> Product/2
  Coolant T (C)/1 -> lambda/1
  HOT fuel use (g/s)/1 -> Product1/1
  Product1/1 -> fuel use (g/s)/1
  CO cold/hot/1 -> Mux/2
  Product/1 -> EO emis (g/s)/1
  fuel cold/hot/1 -> Product1/2
  Mux/1 -> Product/1
  lambda/1 -> Saturation/1
  Saturation/1 -> PM cold/hot/1, NOx cold/hot/1, fuel cold/hot/1, HC cold/hot/1, CO cold/hot/1
  HC cold/hot/1 -> Mux/1
  NOx cold/hot/1 -> Mux/3
  PM cold/hot/1 -> Mux/4

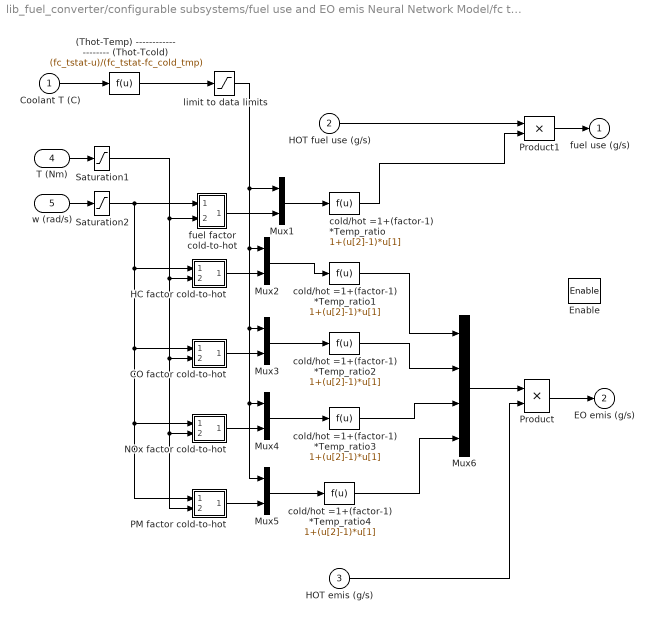
== system lib_fuel_converter/configurable subsystems/fuel use and EO emis Neural Network Model/fc temp correct/fc temp correct Variable Correction Factors (Map Based) ==
  Coolant T (C) : Inport  Port=1  LatchInput=off
  HOT fuel use (g/s) : Inport  Port=2  LatchInput=off
  HOT emis (g/s) : Inport  Port=3  LatchInput=off
  T (Nm) : Inport  Port=4  LatchInput=off
  w (rad/s) : Inport  Port=5  LatchInput=off
  Enable : EnablePort  StatesWhenEnabling=reset
  (Thot-Temp) -------------------- (Thot-Tcold) : Fcn  Expr=(fc_tstat-u)/(fc_tstat-fc_cold_tmp)
  CO factor cold-to-hot : Subsystem  mask(2-D Table Lookup){@1=fc_map_spd*fc_spd_scale, @2=fc_map_trq*fc_trq_scale, @3=fc_co_map_c2h}
      mask prompts: @1 "X Index"; @2 "Y Index"; @3 "Table"
      mask help:
      | Two Dimensional Table Lookup
      | The first input corresponds to X Index and the second input corresponds to the Y Index
      mask init:
      | xindex=@1; yindex=@2; table=@3; sftab2chk(xindex,yindex,table);
      settings: RTWFcnNameOpts=Auto  RTWFileNameOpts=Auto
      mask Help: This block returns a linearly interpolated intersection from the table using the X index (which corresponds to the rows of the table) and the Y index (which corresponds to the columns of the table).  Extrapolation is used.
      mask Display: plot(-10,-10,110,110,[90,50,10],[90,40,30],[90,50,10],[50,26,20],[90,50,10],[22,13,10])
  HC factor cold-to-hot : Subsystem  mask(2-D Table Lookup){@1=fc_map_spd*fc_spd_scale, @2=fc_map_trq*fc_trq_scale, @3=fc_hc_map_c2h}
      mask prompts: @1 "X Index"; @2 "Y Index"; @3 "Table"
      mask help:
      | Two Dimensional Table Lookup
      | The first input corresponds to X Index and the second input corresponds to the Y Index
      mask init:
      | xindex=@1; yindex=@2; table=@3; sftab2chk(xindex,yindex,table);
      settings: RTWFcnNameOpts=Auto  RTWFileNameOpts=Auto
      mask Help: This block returns a linearly interpolated intersection from the table using the X index (which corresponds to the rows of the table) and the Y index (which corresponds to the columns of the table).  Extrapolation is used.
      mask Display: plot(-10,-10,110,110,[90,50,10],[90,40,30],[90,50,10],[50,26,20],[90,50,10],[22,13,10])
  Mux{1..5} (5 alike) : Mux  Inputs=2
      settings: DisplayOption=none
  Mux6 : Mux  Inputs=4
      settings: DisplayOption=none
  NOx factor cold-to-hot : Subsystem  mask(2-D Table Lookup){@1=fc_map_spd*fc_spd_scale, @2=fc_map_trq*fc_trq_scale, @3=fc_nox_map_c2h}
      mask prompts: @1 "X Index"; @2 "Y Index"; @3 "Table"
      mask help:
      | Two Dimensional Table Lookup
      | The first input corresponds to X Index and the second input corresponds to the Y Index
      mask init:
      | xindex=@1; yindex=@2; table=@3; sftab2chk(xindex,yindex,table);
      settings: RTWFcnNameOpts=Auto  RTWFileNameOpts=Auto
      mask Help: This block returns a linearly interpolated intersection from the table using the X index (which corresponds to the rows of the table) and the Y index (which corresponds to the columns of the table).  Extrapolation is used.
      mask Display: plot(-10,-10,110,110,[90,50,10],[90,40,30],[90,50,10],[50,26,20],[90,50,10],[22,13,10])
  PM factor cold-to-hot : Subsystem  mask(2-D Table Lookup){@1=fc_map_spd*fc_spd_scale, @2=fc_map_trq*fc_trq_scale, @3=fc_pm_map_c2h}
      mask prompts: @1 "X Index"; @2 "Y Index"; @3 "Table"
      mask help:
      | Two Dimensional Table Lookup
      | The first input corresponds to X Index and the second input corresponds to the Y Index
      mask init:
      | xindex=@1; yindex=@2; table=@3; sftab2chk(xindex,yindex,table);
      settings: RTWFcnNameOpts=Auto  RTWFileNameOpts=Auto
      mask Help: This block returns a linearly interpolated intersection from the table using the X index (which corresponds to the rows of the table) and the Y index (which corresponds to the columns of the table).  Extrapolation is used.
      mask Display: plot(-10,-10,110,110,[90,50,10],[90,40,30],[90,50,10],[50,26,20],[90,50,10],[22,13,10])
  Product : Product  Inputs=2  Multiplication=Element-wise(.*)  SaturateOnIntegerOverflow=on
  Product1 : Product  Inputs=2  Multiplication=Element-wise(.*)  SaturateOnIntegerOverflow=on
  Saturation1 : Saturate  UpperLimit=max(fc_map_trq*fc_trq_scale)  LowerLimit=min(fc_map_trq*fc_trq_scale)  LinearizeAsGain=on
  Saturation2 : Saturate  UpperLimit=max(fc_map_spd*fc_spd_scale)  LowerLimit=min(fc_map_spd*fc_spd_scale)  LinearizeAsGain=on
  cold/hot =1+(factor-1) *Temp_ratio{,1..4} (5 alike) : Fcn  Expr=1+(u[2]-1)*u[1]
  fuel factor cold-to-hot : Subsystem  mask(2-D Table Lookup){@1=fc_map_spd*fc_spd_scale, @2=fc_map_trq*fc_trq_scale, @3=fc_fuel_map_c2h}
      mask prompts: @1 "X Index"; @2 "Y Index"; @3 "Table"
      mask help:
      | Two Dimensional Table Lookup
      | The first input corresponds to X Index and the second input corresponds to the Y Index
      mask init:
      | xindex=@1; yindex=@2; table=@3; sftab2chk(xindex,yindex,table);
      settings: RTWFcnNameOpts=Auto  RTWFileNameOpts=Auto
      mask Help: This block returns a linearly interpolated intersection from the table using the X index (which corresponds to the rows of the table) and the Y index (which corresponds to the columns of the table).  Extrapolation is used.
      mask Display: plot(-10,-10,110,110,[90,50,10],[90,40,30],[90,50,10],[50,26,20],[90,50,10],[22,13,10])
  limit to data limits : Saturate  UpperLimit=1  LowerLimit=0  LinearizeAsGain=on
  fuel use (g/s) : Outport  Port=1  OutputWhenDisabled=reset  InitialOutput=0
  EO emis (g/s) : Outport  Port=2  OutputWhenDisabled=reset  InitialOutput=0
  wires:
  HOT fuel use (g/s)/1 -> Product1/1
  Saturation2/1 -> fuel factor cold-to-hot/1(x0), HC factor cold-to-hot/1(x0), CO factor cold-to-hot/1(x0), NOx factor cold-to-hot/1(x0), PM factor cold-to-hot/1(x0)
  Saturation1/1 -> fuel factor cold-to-hot/2(y0), HC factor cold-to-hot/2(y0), CO factor cold-to-hot/2(y0), NOx factor cold-to-hot/2(y0), PM factor cold-to-hot/2(y0)
  Coolant T (C)/1 -> (Thot-Temp) -------------------- (Thot-Tcold)/1
  fuel factor cold-to-hot/1(table out) -> Mux1/2
  Mux1/1 -> cold/hot =1+(factor-1) *Temp_ratio/1
  HC factor cold-to-hot/1(table out) -> Mux2/2
  CO factor cold-to-hot/1(table out) -> Mux3/2
  NOx factor cold-to-hot/1(table out) -> Mux4/2
  PM factor cold-to-hot/1(table out) -> Mux5/2
  Mux2/1 -> cold/hot =1+(factor-1) *Temp_ratio1/1
  Mux3/1 -> cold/hot =1+(factor-1) *Temp_ratio2/1
  Mux4/1 -> cold/hot =1+(factor-1) *Temp_ratio3/1
  Mux5/1 -> cold/hot =1+(factor-1) *Temp_ratio4/1
  Product1/1 -> fuel use (g/s)/1
  Product/1 -> EO emis (g/s)/1
  HOT emis (g/s)/1 -> Product/2
  T (Nm)/1 -> Saturation1/1
  w (rad/s)/1 -> Saturation2/1
  Mux6/1 -> Product/1
  (Thot-Temp) -------------------- (Thot-Tcold)/1 -> limit to data limits/1
  limit to data limits/1 -> Mux1/1, Mux2/1, Mux3/1, Mux4/1, Mux5/1
  cold/hot =1+(factor-1) *Temp_ratio/1 -> Product1/2
  cold/hot =1+(factor-1) *Temp_ratio1/1 -> Mux6/1
  cold/hot =1+(factor-1) *Temp_ratio2/1 -> Mux6/2
  cold/hot =1+(factor-1) *Temp_ratio3/1 -> Mux6/3
  cold/hot =1+(factor-1) *Temp_ratio4/1 -> Mux6/4

== system lib_fuel_converter/fuel converter  <fc>/engine speed estimator/no-lag Reset Integrator/dt ==
  Clock : Clock
      settings: DisplayTime=off  Decimation=10
  Memory1 : Memory  X0=-0.1  InheritSampleTime=off
      settings: RTWStateStorageClass=Auto
  Sum1 : Sum  Inputs=+-  SaturateOnIntegerOverflow=on
  out_1 : Outport  Port=1  InitialOutput=0
  wires:
  Clock/1 -> Sum1/1, Memory1/1
  Memory1/1 -> Sum1/2
  Sum1/1 -> out_1/1

== system lib_fuel_converter/fuel converter  <fc>/engine torque/effect of inertia (Nm)/Block NOTES ==
  note: Torque required to accelerate the engine inertia is taken from the engine
      | acceleration, and is assumed to be no less than zero if the trace was missed
      | at all on the previous time step.
      |
      | The torque required to accelerate the engine's inertia is never assumed to
      | be more than the product of the engine's maximum torque and the engine's
      | contribution to the total vehicle inertia.

== system lib_fuel_converter/fuel converter  <fc> for series/providing trq (+ive or -ive)/enforce engine limits/Block NOTES ==
  note: This block enforces performance limits on torque and speed.  At no time will
      | engine torque be greater than its capability or less than its closed-throttle torque.
      | If the engine is in free spindown, the engine torque used for fuel use computation
      | is the closed-throttle torque.  At no time will engine speed be greater than its
      | maximum (safe) speed or less than idle speed if idling or zero if off.  During spindown,
      | engine speed is calculated using engine inertia and the drag torques on the engine.

== system lib_fuel_converter/fuel converter  <fc> for series/providing trq (+ive or -ive)/enforce engine limits/T_closed throttle ==
  w_APU : Inport  Port=1  LatchInput=off
  Saturation : Saturate  UpperLimit=max(fc_map_spd)*fc_spd_scale  LowerLimit=min(fc_map_spd)*fc_spd_scale  LinearizeAsGain=on
  ctt lookup : Lookup  InputValues=fc_map_spd*fc_spd_scale  OutputValues=fc_ct_trq*fc_trq_scale
  T_closed throttle : Outport  Port=1  InitialOutput=0
  wires:
  ctt lookup/1 -> T_closed throttle/1
  Saturation/1 -> ctt lookup/1
  w_APU/1 -> Saturation/1

== system lib_fuel_converter/fuel converter  <fc> for series/providing trq (+ive or -ive)/enforce engine limits/T_max ==
  w_APU : Inport  Port=1  LatchInput=off
  Saturation1 : Saturate  UpperLimit=max(fc_map_spd)*fc_spd_scale  LowerLimit=min(fc_map_spd)*fc_spd_scale  LinearizeAsGain=on
  max_torque lookup : Lookup  InputValues=fc_map_spd*fc_spd_scale  OutputValues=fc_max_trq*fc_trq_scale
  T_max : Outport  Port=1  InitialOutput=0
  wires:
  Saturation1/1 -> max_torque lookup/1
  w_APU/1 -> Saturation1/1
  max_torque lookup/1 -> T_max/1

== system lib_fuel_converter/fuel converter  <fc> for series/spinning up or spinning down/no-lag Reset Integrator/dt ==
  Clock : Clock
      settings: DisplayTime=off  Decimation=10
  Memory1 : Memory  X0=-0.1  InheritSampleTime=off
      settings: RTWStateStorageClass=Auto
  Sum1 : Sum  Inputs=+-  SaturateOnIntegerOverflow=on
  out_1 : Outport  Port=1  InitialOutput=0
  wires:
  Clock/1 -> Sum1/1, Memory1/1
  Memory1/1 -> Sum1/2
  Sum1/1 -> out_1/1

== system lib_fuel_converter/fuel converter  <fc> prius/providing trq (+ive or -ive)/accessories (Nm)/key_on ==
  Clock : Clock
      settings: DisplayTime=off  Decimation=10
  Fcn1 : Fcn  Expr=rem(u[1],period)
  Look-Up Table : Lookup  InputValues=t  OutputValues=y
  out_1 : Outport  Port=1  InitialOutput=0
  wires:
  Fcn1/1 -> Look-Up Table/1
  Clock/1 -> Fcn1/1
  Look-Up Table/1 -> out_1/1

== system lib_fuel_converter/fuel converter  <fc> prius/providing trq (+ive or -ive)/enforce engine limits/Block NOTES ==
  note: This block enforces performance limits on torque and speed.  At no time will
      | engine torque be greater than its capability or less than its closed-throttle torque.
      | If the engine is in free spindown, the engine torque used for fuel use computation
      | is the closed-throttle torque.  At no time will engine speed be greater than its
      | maximum (safe) speed or less than idle speed if idling or zero if off.  During spindown,
      | engine speed is calculated using engine inertia and the drag torques on the engine.

== system lib_fuel_converter/fuel converter  <fc> prius/providing trq (+ive or -ive)/enforce engine limits/T_closed throttle ==
  w_APU : Inport  Port=1  LatchInput=off
  Saturation : Saturate  UpperLimit=max(fc_map_spd)*fc_spd_scale  LowerLimit=min(fc_map_spd)*fc_spd_scale  LinearizeAsGain=on
  ctt lookup : Lookup  InputValues=fc_map_spd*fc_spd_scale  OutputValues=fc_ct_trq*fc_trq_scale
  T_closed throttle : Outport  Port=1  InitialOutput=0
  wires:
  w_APU/1 -> Saturation/1
  Saturation/1 -> ctt lookup/1
  ctt lookup/1 -> T_closed throttle/1

== system lib_fuel_converter/fuel converter  <fc> prius/providing trq (+ive or -ive)/enforce engine limits/T_max ==
  w_APU : Inport  Port=1  LatchInput=off
  Saturation1 : Saturate  UpperLimit=max(fc_map_spd)*fc_spd_scale  LowerLimit=min(fc_map_spd)*fc_spd_scale  LinearizeAsGain=on
  max_torque lookup : Lookup  InputValues=fc_map_spd*fc_spd_scale  OutputValues=fc_max_trq*fc_trq_scale
  T_max : Outport  Port=1  InitialOutput=0
  wires:
  max_torque lookup/1 -> T_max/1
  w_APU/1 -> Saturation1/1
  Saturation1/1 -> max_torque lookup/1

== system lib_fuel_converter/configurable subsystems/fuel use and EO emis/fc temp/fc mass heat flow/Block NOTES ==
  note: FUEL CONVERTER MASS HEAT LOSS
      | This block models the heat loss from a fuel converter (such as an IC engine).
      | Convection (as a function of vehicle speed), radiation, and conduction effects are included.
      | Engine cylinder (c), interior (i), exterior (x) and hood (h)
      | heat flows are estimated based on the temperatures from the previous iteration.

== system lib_fuel_converter/configurable subsystems/fuel use and EO emis/fc temp/old fc coolant  temp. (C)/Block NOTES ==
  note: This block computes engine coolant temperature,
      | assuming that it asymptotically approaches its maximum
      | temperature when the engine is on, and asymptotically
      | approaches the ambient temperature when the engine
      | is off.  Temperatue rise rate is assumed to be a function
      | only of current engine coolant temperature, and the fall
      | rate is also a function of vehicle speed and ambient temperature.
      | There is no dependence on engine load or speed.

== system lib_fuel_converter/configurable subsystems/fuel use and EO emis/fc temp correct/fc temp correct Constant Correction Factors (Equation Based)/Block NOTES ==
  note: This block determines actual fuel use and engine-out emissions
      | given the fully hot values and the engine coolant temperature.
      | The correlations used here were developed at NREL using
      | Hot and Cold Engine data collected
      | at Oak Ridge National Laboratory.
